simulink model "dcdc_2017b"  (Simulink 9.0)
settings: Solver=VariableStepAuto  StartTime=0.0  StopTime=0.4  FixedStep=t_step  MaxStep=1e-6  RelTol=1e-3
values from neighbouring files (symbols this model uses):
  Cb = 100e-6    (= 0.0001)    [params.m]
  Lb = 1e-3    (= 0.001)    [params.m]
undefined symbols (not defined in the file or in its folder): Ion, Lithium, t_step
libraries: powerlib x17, powerlib_meascontrol x4, electricdrivelib x1
settings Model: Creator=Chuanyue Li  LastModifiedBy=c2107789
settings SolverCC: ZeroCrossAlgorithm=Adaptive
settings DataIOCC: SaveFormat=Dataset
settings OptimizationCC: LifeSpan=auto
settings DebuggingCC: UnderspecifiedInitializationDetection=Simplified  MergeDetectMultiDrivingBlocksExec=error  IgnoredZcDiagnostic=none  SFUnexpectedBacktrackingDiag=error  SFNoUnconditionalDefaultTransitionDiag=error  SFExecutionAtInitializationDiag=warning
settings HardwareCC: ProdBitPerPointer=64  ProdBitPerSizeT=64  ProdBitPerPtrDiffT=64  ProdLargestAtomicFloat=Float  ProdIntDivRoundTo=Zero  ProdEndianess=LittleEndian  ProdWordSize=64  ProdHWDeviceType=Intel->x86-64 (Windows64)
settings ModelReferenceCC: PropagateSignalLabelsOutOfModel=on
settings CodeAppCC: StateflowObjectComments=off
settings GRTTargetCC: TargetLangStandard=C99 (ISO)
settings ConfigComp: CovMetricSettings=dwe  CovSaveCumulativeToWorkspaceVar=off  CovSaveSingleToWorkspaceVar=off  CovExternalEMLEnable=on

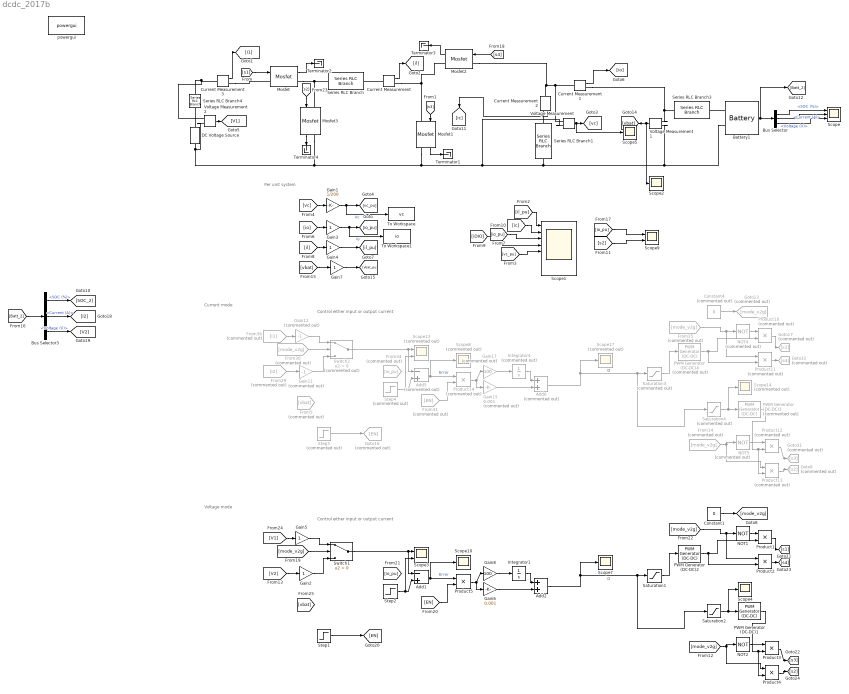
== system dcdc_2017b ==
  note: Per unit system
  note: Control either input or output current
  note: Current mode
  note: Control either input or output current
  note: Voltage mode
  Add1 : Sum  Inputs=-+
  Add2 : Sum
  Add5 : Sum  Commented=on  Inputs=-+
  Add6 : Sum  Commented=on
  Battery1 : electricdrivelib/Extra Sources/Battery  BatType=Lithium-Ion  ShowTempParam=off  ThermalPreset=no  ShowAgeParam=off  NomV=380  NomQ=500  SOC=69.98  Batt_Tr=1  PresetModel=on  MaxQ=500  MinV=285  FullV=442.3151  Dis_rate=217.3913  R=0.0076  Normal_OP=452.1739  expZone="[410.5466      24.56522]"  current=[6.5 13 32.5]  Units=Time  Tci=20  NomT=20  T2=-30  MaxQ2=4.8  FullV2=7.1  Normal_OP2=5.655  expZone2="[6.58           1]"  Rca=0.6  ti=2000  Dp=0  Neq0=0  Tsim=1e6  Ta1=25  Qeol=5.4*0.9  Reol=0.013333*1.2  Char_age=[2.3478, 3]  Dis_age=[2.3478, 10]  N1=1500  N2=10500  N3=1000  N4=1400  Ta2=45  N5=950
  Bus Selector : BusSelector  OutputSignals=SOC (%),Current (A),Voltage (V)
  Bus Selector3 : BusSelector  OutputSignals=SOC (%),Current (A),Voltage (V)
  Constant1 : Constant  Value=0
  Constant4 : Constant  Commented=on  Value=0
  Current Measurement{,1..3} (4 alike) : powerlib/Measurements/Current Measurement  PhasorSimulation=off  OutputType=Complex  PSBequivalent=0
  DC Voltage Source : powerlib/Electrical Sources/DC Voltage Source  Amplitude=415  Measurements=None
  From14 : From  Commented=on  GotoTag=mode_v2g
  From29 : From  Commented=on  GotoTag=I2
  From30 : From  Commented=on  GotoTag=mode_v2g
  From31 : From  Commented=on  GotoTag=EN
  From34 : From  Commented=on  GotoTag=io_pu
  From35 : From  Commented=on  GotoTag=mode_v2g
  From36 : From  Commented=on  GotoTag=I1
  From5 : From  Commented=on  GotoTag=vbat
  Gain1 : Gain  Gain=1/200
  Gain11 : Gain  Commented=on  Gain=-1
  Gain12 : Gain  Commented=on  Gain=-1
  Gain15 : Gain  Commented=on  Gain=0.001
  Gain17 : Gain  Commented=on  Gain=100
  Gain{2..5,7} (5 alike) : Gain
  Gain6 : Gain  Gain=0.001
  Gain8 : Gain  Gain=100
  Goto13 : Goto  Commented=on  GotoTag=mode_v2g
  Goto16 : Goto  Commented=on  GotoTag=EN
  Goto17 : Goto  Commented=on  GotoTag=s1
  Goto31 : Goto  Commented=on  GotoTag=s3
  Goto32 : Goto  Commented=on  GotoTag=s4
  Goto9 : Goto  Commented=on  GotoTag=s2
  Integrator1 : Integrator  LimitOutput=on  UpperSaturationLimit=1  LowerSaturationLimit=0
  Integrator4 : Integrator  Commented=on  LimitOutput=on  UpperSaturationLimit=1  LowerSaturationLimit=0
  Mosfet : powerlib/Power Electronics/Mosfet  Ron=0.1  Lon=0  Rd=0.01  Vfd=0  IC=0  Rs=1e5  Cs=inf  Measurements=on
  Mosfet1 : powerlib/Power Electronics/Mosfet  Ron=0.01  Lon=0  Rd=0.01  Vfd=0  IC=0  Rs=1e5  Cs=inf  Measurements=on
  Mosfet2 : powerlib/Power Electronics/Mosfet  Ron=0.1  Lon=0  Rd=0.01  Vfd=0  IC=0  Rs=1e5  Cs=inf  Measurements=on
  Mosfet3 : powerlib/Power Electronics/Mosfet  Ron=0.1  Lon=0  Rd=0.01  Vfd=0  IC=0  Rs=1e5  Cs=inf  Measurements=on
  NOT1 : Logic  Operator=NOT  IconShape=distinctive  AllPortsSameDT=off  OutDataTypeStr=boolean
  NOT2 : Logic  Operator=NOT  IconShape=distinctive  AllPortsSameDT=off  OutDataTypeStr=boolean
  NOT4 : Logic  Commented=on  Operator=NOT  IconShape=distinctive  AllPortsSameDT=off  OutDataTypeStr=boolean
  NOT5 : Logic  Commented=on  Operator=NOT  IconShape=distinctive  AllPortsSameDT=off  OutDataTypeStr=boolean
  PWM Generator (DC-DC)1 : powerlib_meascontrol/Pulse & Signal Generators/PWM Generator (DC-DC)  Fsw=s_fre  Ts=0
  PWM Generator (DC-DC)2 : powerlib_meascontrol/Pulse & Signal Generators/PWM Generator (DC-DC)  Fsw=s_fre  Ts=0
  PWM Generator (DC-DC)3 : powerlib_meascontrol/Pulse & Signal Generators/PWM Generator (DC-DC)  Commented=on  Fsw=s_fre  Ts=0
  PWM Generator (DC-DC)4 : powerlib_meascontrol/Pulse & Signal Generators/PWM Generator (DC-DC)  Commented=on  Fsw=s_fre  Ts=0
  Product{1..5} (5 alike) : Product
  Product{10..14} (5 alike) : Product  Commented=on
  Saturation1 : Saturate  UpperLimit=0.95  LowerLimit=0
  Saturation2 : Saturate  UpperLimit=0.8  LowerLimit=0
  Saturation3 : Saturate  Commented=on  UpperLimit=0.95  LowerLimit=0
  Saturation4 : Saturate  Commented=on  UpperLimit=0.8  LowerLimit=0
  Scope : Scope  NumInputPorts=3
  Scope1 : Scope  NumInputPorts=8
  Scope{2,4..5,7,10} (5 alike) : Scope
  Scope13 : Scope  Commented=on  NumInputPorts=2
  Scope14 : Scope  Commented=on
  Scope17 : Scope  Commented=on
  Scope3 : Scope  NumInputPorts=2
  Scope8 : Scope  Commented=on
  Scope9 : Scope  NumInputPorts=2
  Series RLC Branch : powerlib/Elements/Series RLC Branch  LConnTagsString=__new0  RConnTagsString=__new0  BranchType=L  Resistance=1  Inductance=Lb/100  SetiL0=off  InitialCurrent=0  Capacitance=1e-6  Setx0=off  InitialVoltage=0  Measurements=None
  Series RLC Branch1 : powerlib/Elements/Series RLC Branch  LConnTagsString=__new0  RConnTagsString=__new0  BranchType=C  Resistance=1  Inductance=1e-3  SetiL0=off  InitialCurrent=0  Capacitance=Cb  Setx0=off  InitialVoltage=0  Measurements=None
  Series RLC Branch3 : powerlib/Elements/Series RLC Branch  LConnTagsString=__new0  RConnTagsString=__new0  BranchType=R  Resistance=1  Inductance=1e-3  SetiL0=off  InitialCurrent=0  Capacitance=Cb  Setx0=off  InitialVoltage=0  Measurements=None
  Series RLC Branch4 : powerlib/Elements/Series RLC Branch  LConnTagsString=__new0  RConnTagsString=__new0  BranchType=R  Resistance=1e-3  Inductance=1e-3  SetiL0=off  InitialCurrent=0  Capacitance=Cb  Setx0=off  InitialVoltage=0  Measurements=None
  Step1 : Step  Time=0.025  SampleTime=0
  Step2 : Step  Time=0.2  Before=412  After=413  SampleTime=0
  Step3 : Step  Commented=on  Time=0.025  SampleTime=0
  Step4 : Step  Commented=on  Before=25  After=11  SampleTime=0
  Switch1 : Switch  Criteria=u2 > Threshold
  Switch2 : Switch  Commented=on  Criteria=u2 > Threshold
  Terminator{1..4} (4 alike) : Terminator
  To Workspace : ToWorkspace  VariableName=vc  SaveFormat=Timeseries  SampleTime=-1
  To Workspace1 : ToWorkspace  VariableName=io  SaveFormat=Timeseries  SampleTime=-1
  Voltage Measurement : powerlib/Measurements/Voltage Measurement  PhasorSimulation=off  OutputType=Complex  PSBequivalent=0
  Voltage Measurement1 : powerlib/Measurements/Voltage Measurement  PhasorSimulation=off  OutputType=Complex  PSBequivalent=0
  Voltage Measurement2 : powerlib/Measurements/Voltage Measurement  PhasorSimulation=off  OutputType=Complex  PSBequivalent=0
  powergui : powerlib/powergui  Priority=1  SimulationMode=Continuous  SampleTime=t_step*10  frequency=60  Iterations=50  frequencyindice=0  Pbase=100e6  ErrMax=1e-4  UnitsV=kV  UnitsW=MW  buscounter=0  FunctionMessages=off  echomessages=off  EnableUseOfTLC=off  CurrentSourceSwitches=off  DisableSnubberDevices=off  DisableRonSwitches=off  DisableVfSwitches=off  DisplayEquations=off  AutomaticDiscreteSolvers=off  SolverType=Tustin/Backward Euler (TBE)  Interpol=off  ExternalGateDelay=off  methode=off  Ts=100  x0status=blocks  SPID=off  SwTol=0  HookPort=off  NonlinearTolerance=1e-4  nMaxIteration=100  ContinueOnMaxIteration=off  RestoreLinks=warning  ResistiveCurrentMeasurement=off  Frange=[0:2:500]  Ylog=off  Xlog=on  ShowGrid=off  save=off  variable=ZData  structure=0  ZoomFFT=off  StartTime=0.0  cycles=1  DisplayStyle=1  fundamental=60  FreqAxis=off  MaxFrequency=1000  frequencyindicesteady=1  RmsSteady=1  display=off
  wires:
  [s1] -> Mosfet/1
  [s3] -> Mosfet1/1
  Current Measurement/1 -> [il]
  Voltage Measurement/1 -> Scope5/1, [vc]
  [il_pu] -> Scope1/1
  [vc] -> Gain1/1
  Gain1/1 -> To Workspace/1, [vc_pu]  "Vc"
  Bus Selector/1 -> Scope/1  "<SOC (%)>"
  Bus Selector/2 -> Scope/2  "<Current (A)>"
  Bus Selector/3 -> Scope/3  "<Voltage (V)>"
  [io] -> Gain3/1
  Current Measurement1/1 -> [io]
  Gain3/1 -> To Workspace1/1, [io_pu]  "Io"
  [io_pu] -> Scope1/3
  Gain4/1 -> [il_pu]
  [il] -> Gain4/1
  [iDIO] -> Scope1/4
  Current Measurement2/1 -> [ic]
  [ic] -> Scope1/2
  [vc_pu] -> Scope1/5
  Voltage Measurement1/1 -> Scope2/1, [vbat]
  [vbat] -> Gain7/1
  Gain7/1 -> [vbat_pu]
  Mosfet1/1 -> Terminator1/1
  Mosfet/1 -> Terminator2/1
  [io_pu] -> Scope9/1
  [s2] -> Scope9/2
  Mosfet2/1 -> Terminator3/1
  [s4] -> Mosfet2/1
  [s2] -> Mosfet3/1
  Mosfet3/1 -> Terminator4/1
  Battery1/1 -> [Batt_2], Bus Selector/1
  [Batt_2] -> Bus Selector3/1
  Bus Selector3/3 -> [V2]  "<Voltage (V)>"
  Bus Selector3/2 -> [I2]  "<Current (A)>"
  Bus Selector3/1 -> [SOC_2]  "<SOC (%)>"
  Current Measurement3/1 -> [I1]
  Voltage Measurement2/1 -> [V1]
  From36/1 -> Gain12/1
  Gain12/1 -> Switch2/1
  Gain11/1 -> Switch2/3
  NOT5/1 -> Product12/1
  NOT4/1 -> Product10/1
  Saturation3/1 -> PWM Generator (DC-DC)4/1
  Integrator4/1 -> Add6/1
  Add6/1 -> Saturation4/1, Saturation3/1, Scope17/1  "D"
  From31/1 -> Product14/2
  Product14/1 -> Gain17/1, Gain15/1
  Step3/1 -> Goto16/1
  Gain15/1 -> Add6/2
  Gain17/1 -> Integrator4/1
  Step4/1 -> Scope13/2, Add5/2
  Add5/1 -> Product14/1, Scope8/1  "Error"
  Saturation4/1 -> PWM Generator (DC-DC)3/1, Scope14/1
  PWM Generator (DC-DC)4/1 -> Product10/2, Product11/2
  From29/1 -> Gain11/1
  From30/1 -> Switch2/2
  Product10/1 -> Goto17/1
  Product11/1 -> Goto32/1
  From35/1 -> Product11/1, NOT4/1
  From14/1 -> NOT5/1, Product13/1
  Product13/1 -> Goto9/1
  Product12/1 -> Goto31/1
  PWM Generator (DC-DC)3/1 -> Product13/2, Product12/2
  Constant4/1 -> Goto13/1
  Switch2/1 -> Add5/1, Scope13/1
  Switch1/1 -> Scope3/1, Add1/1
  Constant1/1 -> [mode_v2g]
  PWM Generator (DC-DC)1/1 -> Product3/2, Product4/2
  Product3/1 -> [s3]
  Product4/1 -> [s2]
  [mode_v2g] -> Product4/1, NOT2/1
  [mode_v2g] -> NOT1/1, Product2/1
  Product2/1 -> [s4]
  Product1/1 -> [s1]
  [mode_v2g] -> Switch1/2
  [V2] -> Gain2/1
  PWM Generator (DC-DC)2/1 -> Product2/2, Product1/2
  Saturation2/1 -> Scope4/1, PWM Generator (DC-DC)1/1
  Add1/1 -> Scope10/1, Product5/1  "Error"
  Step2/1 -> Add1/2, Scope3/2
  Gain8/1 -> Integrator1/1
  Gain6/1 -> Add2/2
  Step1/1 -> [EN]
  Product5/1 -> Gain6/1, Gain8/1
  [EN] -> Product5/2
  Add2/1 -> Scope7/1, Saturation1/1, Saturation2/1  "D"
  Integrator1/1 -> Add2/1
  Saturation1/1 -> PWM Generator (DC-DC)2/1
  NOT1/1 -> Product1/1
  NOT2/1 -> Product3/1
  Gain2/1 -> Switch1/3
  Gain5/1 -> Switch1/1
  [V1] -> Gain5/1
  connections:
  Mosfet/RConn1 -- Mosfet3/LConn1 -- Series RLC Branch/LConn1
  Current Measurement/LConn1 -- Series RLC Branch/RConn1
  Current Measurement2/RConn1 -- Series RLC Branch1/LConn1
  Battery1/LConn2 -- Voltage Measurement/LConn2 -- Voltage Measurement2/LConn2 -- DC Voltage Source/LConn1 -- Mosfet3/RConn1 -- Mosfet1/RConn1 -- Series RLC Branch1/RConn1 -- Voltage Measurement1/LConn2
  Mosfet1/LConn1 -- Mosfet2/RConn1 -- Current Measurement/RConn1
  DC Voltage Source/RConn1 -- Series RLC Branch4/RConn1
  Current Measurement3/RConn1 -- Mosfet/LConn1
  Series RLC Branch4/LConn1 -- Voltage Measurement2/LConn1 -- Current Measurement3/LConn1
  Current Measurement1/LConn1 -- Voltage Measurement/LConn1 -- Mosfet2/LConn1 -- Current Measurement2/LConn1
  Voltage Measurement1/LConn1 -- Current Measurement1/RConn1 -- Series RLC Branch3/RConn1
  Battery1/LConn1 -- Series RLC Branch3/LConn1
